simulink model "fir_model"  (R2015a)
settings: Solver=ode3  StartTime=0.0  StopTime=10  FixedStep=0.0033  RelTol=1e-3
settings Model: Creator=Diana German  LastModifiedBy=Diana German

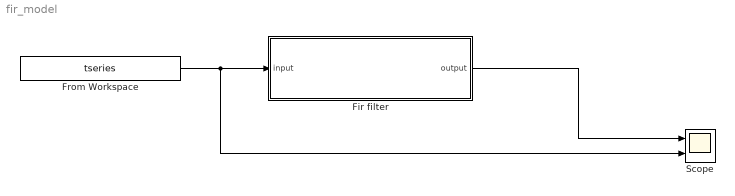
== system fir_model ==
  Fir filter : Subsystem
  From Workspace : FromWorkspace  VariableName=tseries  SampleTime=0
  Scope : Scope  NumInputPorts=2
      settings: ShowLegends=on  YMin=-5~-5  YMax=5~5
  wires:
  Fir filter/1(output) -> Scope/1
  From Workspace/1 -> Scope/2, Fir filter/1(input)

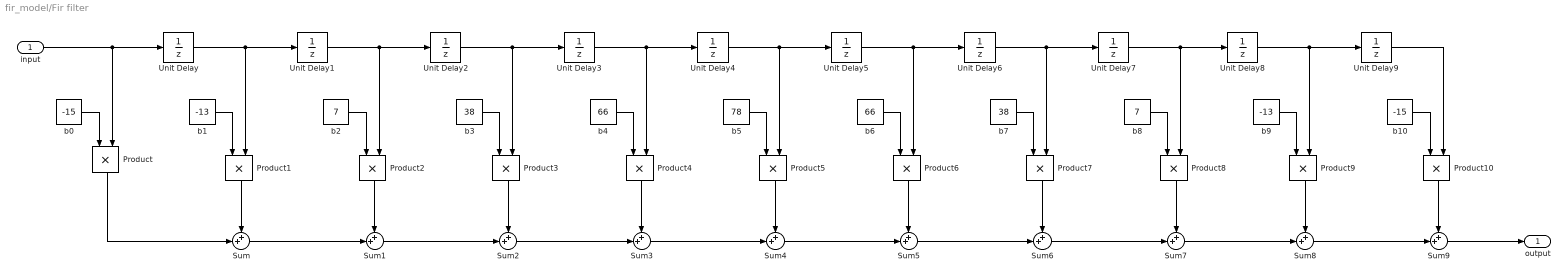
== system fir_model/Fir filter ==
  input : Inport
  Product{,1..10} (11 alike) : Product
  Sum{,1..9} (10 alike) : Sum  Inputs=++|
  Unit Delay{,1..9} (10 alike) : UnitDelay  SampleTime=-1
  b0 : Constant  Value=-15
  b1 : Constant  Value=-13
  b10 : Constant  Value=-15
  b2 : Constant  Value=7
  b3 : Constant  Value=38
  b4 : Constant  Value=66
  b5 : Constant  Value=78
  b6 : Constant  Value=66
  b7 : Constant  Value=38
  b8 : Constant  Value=7
  b9 : Constant  Value=-13
  output : Outport
  wires:
  input/1 -> Product/2, Unit Delay/1
  b0/1 -> Product/1
  Sum/1 -> Sum1/2
  Unit Delay/1 -> Unit Delay1/1, Product1/2
  b1/1 -> Product1/1
  Product1/1 -> Sum/1
  Product2/1 -> Sum1/1
  b2/1 -> Product2/1
  Product/1 -> Sum/2
  Unit Delay1/1 -> Unit Delay2/1, Product2/2
  Product3/1 -> Sum2/1
  Sum1/1 -> Sum2/2
  b3/1 -> Product3/1
  Sum2/1 -> Sum3/2
  Unit Delay2/1 -> Unit Delay3/1, Product3/2
  Product4/1 -> Sum3/1
  b4/1 -> Product4/1
  Sum3/1 -> Sum4/2
  Unit Delay3/1 -> Unit Delay4/1, Product4/2
  Product5/1 -> Sum4/1
  b5/1 -> Product5/1
  Sum4/1 -> Sum5/2
  Unit Delay4/1 -> Unit Delay5/1, Product5/2
  Product6/1 -> Sum5/1
  b6/1 -> Product6/1
  Sum5/1 -> Sum6/2
  Unit Delay5/1 -> Unit Delay6/1, Product6/2
  Product7/1 -> Sum6/1
  b7/1 -> Product7/1
  Sum6/1 -> Sum7/2
  Unit Delay6/1 -> Unit Delay7/1, Product7/2
  Product8/1 -> Sum7/1
  b8/1 -> Product8/1
  Sum7/1 -> Sum8/2
  Unit Delay7/1 -> Unit Delay8/1, Product8/2
  Product9/1 -> Sum8/1
  b9/1 -> Product9/1
  Sum8/1 -> Sum9/2
  Unit Delay8/1 -> Unit Delay9/1, Product9/2
  Product10/1 -> Sum9/1
  b10/1 -> Product10/1
  Unit Delay9/1 -> Product10/2
  Sum9/1 -> output/1
